simulink model "FruitSorting_Hardware"  (R2025a)
settings: Solver=FixedStepDiscrete  StartTime=0.0  StopTime=30  FixedStep=0.05  RelTol=1e-3
undefined symbols (not defined in the file or in its folder): DiscIntNeverNeededParam
settings Model: Creator=Mugin  LastModifiedBy=Mugin

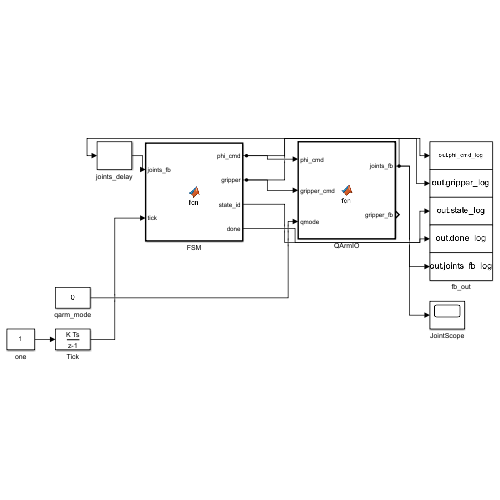
[thumbnail: Simulink's stored preview of the top-level diagram]
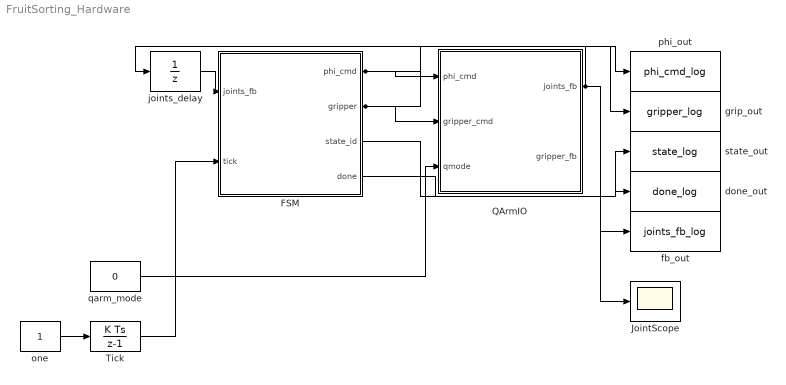
== system FruitSorting_Hardware ==
  FSM : MATLAB Function  TreatAsAtomicUnit=on
  JointScope : Scope
  QArmIO : MATLAB Function  TreatAsAtomicUnit=on
  Tick : DiscreteIntegrator  gainval=1  SampleTime=0.05  ICPrevOutput=DiscIntNeverNeededParam  ICPrevScaledInput=DiscIntNeverNeededParam
  done_out : ToWorkspace  VariableName=done_log  SampleTime=-1
  fb_out : ToWorkspace  VariableName=joints_fb_log  SampleTime=-1
  grip_out : ToWorkspace  VariableName=gripper_log  SampleTime=-1
  joints_delay : UnitDelay  InitialCondition=[0;0;0;0]  SampleTime=0.05  HasFrameUpgradeWarning=on
  one : Constant  SampleTime=0.05
  phi_out : ToWorkspace  VariableName=phi_cmd_log  SampleTime=-1
  qarm_mode : Constant  Value=0  OutDataTypeStr=int32  SampleTime=0.05
  state_out : ToWorkspace  VariableName=state_log  SampleTime=-1
  wires:
  one/1 -> Tick/1
  joints_delay/1 -> FSM/1(joints_fb)
  Tick/1 -> FSM/2(tick)
  FSM/1(phi_cmd) -> QArmIO/1(phi_cmd), phi_out/1
  FSM/2(gripper) -> QArmIO/2(gripper_cmd), grip_out/1
  qarm_mode/1 -> QArmIO/3(qmode)
  QArmIO/1(joints_fb) -> joints_delay/1, fb_out/1, JointScope/1
  FSM/3(state_id) -> state_out/1
  FSM/4(done) -> done_out/1

== matlab function FruitSorting_Hardware/QArmIO ==
  data: phi_cmd input; joints_fb output; gripper_cmd input; qmode input; gripper_fb output
function [joints_fb, gripper_fb] = fcn(phi_cmd, gripper_cmd, qmode)
%#codegen
coder.extrinsic('py_qarm_io');
joints_fb = zeros(4,1);
gripper_fb = 0;
[jtmp, gtmp] = py_qarm_io(phi_cmd, gripper_cmd, double(qmode));
joints_fb = double(jtmp);
gripper_fb = double(gtmp);
end

== matlab function FruitSorting_Hardware/FSM ==
  data: joints_fb input; phi_cmd output; tick input; gripper output; state_id output; done output
function [phi_cmd, gripper, state_id, done] = fcn(joints_fb, tick)
%#codegen
coder.extrinsic('py_controller');
phi_cmd = zeros(4,1);
gripper = 0;
state_id = int32(0);
done = int32(0);
reset_flag = double(tick == 0);
[phi_tmp, g_tmp, s_tmp, d_tmp] = py_controller(joints_fb, 0.0500, reset_flag);
phi_cmd = double(phi_tmp);
gripper = double(g_tmp);
state_id = int32(s_tmp);
done = int32(d_tmp);
end
